simulink model "LAB_Triggred_SubSystem"  (R2024b)
settings: Solver=VariableStepAuto  StartTime=0.0  StopTime=10.0  RelTol=1e-3
settings Model: Creator=Ahmad  LastModifiedBy=Ahmad

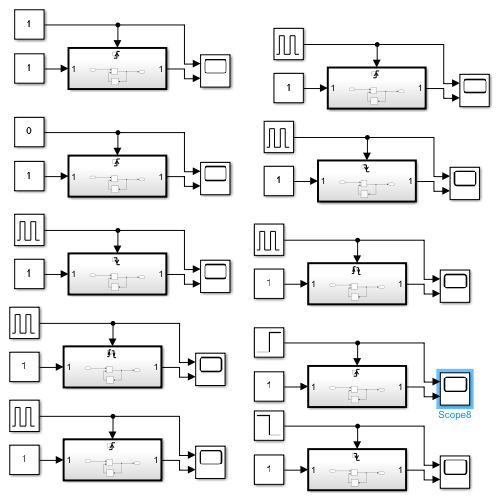
[thumbnail: Simulink's stored preview of the top-level diagram]
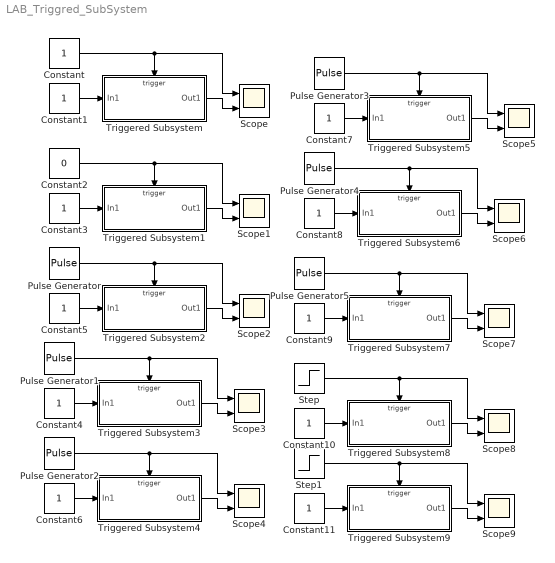
== system LAB_Triggred_SubSystem ==
  Constant{,1,3..11} (11 alike) : Constant
  Constant2 : Constant  Value=0
  Pulse Generator : DiscretePulseGenerator  PulseType=Time based  Period=10  PulseWidth=5
  Pulse Generator1 : DiscretePulseGenerator  PulseType=Time based  Amplitude=5  Period=10  PulseWidth=50
  Pulse Generator2 : DiscretePulseGenerator  PulseType=Time based  Amplitude=10  Period=10  PulseWidth=50  PhaseDelay=2
  Pulse Generator3 : DiscretePulseGenerator  PulseType=Time based  Amplitude=10  Period=1  PulseWidth=10
  Pulse Generator4 : DiscretePulseGenerator  PulseType=Time based  Amplitude=10  Period=1  PulseWidth=10
  Pulse Generator5 : DiscretePulseGenerator  PulseType=Time based  Amplitude=10  Period=1  PulseWidth=10
  Scope{,1..9} (10 alike) : Scope  NumInputPorts=2
  Step : Step  SampleTime=0
  Step1 : Step  Before=1  After=0  SampleTime=0
  Triggered Subsystem : Subsystem  TreatAsAtomicUnit=on
  Triggered Subsystem1 : Subsystem  TreatAsAtomicUnit=on
  Triggered Subsystem2 : Subsystem  TreatAsAtomicUnit=on
  Triggered Subsystem3 : Subsystem  TreatAsAtomicUnit=on
  Triggered Subsystem4 : Subsystem  TreatAsAtomicUnit=on
  Triggered Subsystem5 : Subsystem  TreatAsAtomicUnit=on
  Triggered Subsystem6 : Subsystem  TreatAsAtomicUnit=on
  Triggered Subsystem7 : Subsystem  TreatAsAtomicUnit=on
  Triggered Subsystem8 : Subsystem  TreatAsAtomicUnit=on
  Triggered Subsystem9 : Subsystem  TreatAsAtomicUnit=on
  wires:
  Constant/1 -> Scope/1, Triggered Subsystem/Trigger
  Constant1/1 -> Triggered Subsystem/1(In1)
  Triggered Subsystem/1(Out1) -> Scope/2
  Constant3/1 -> Triggered Subsystem1/1(In1)
  Constant2/1 -> Scope1/1, Triggered Subsystem1/Trigger
  Triggered Subsystem1/1(Out1) -> Scope1/2
  Pulse Generator/1 -> Scope2/1, Triggered Subsystem2/Trigger
  Triggered Subsystem2/1(Out1) -> Scope2/2
  Constant5/1 -> Triggered Subsystem2/1(In1)
  Pulse Generator1/1 -> Scope3/1, Triggered Subsystem3/Trigger
  Constant4/1 -> Triggered Subsystem3/1(In1)
  Triggered Subsystem3/1(Out1) -> Scope3/2
  Triggered Subsystem4/1(Out1) -> Scope4/2
  Constant6/1 -> Triggered Subsystem4/1(In1)
  Pulse Generator2/1 -> Scope4/1, Triggered Subsystem4/Trigger
  Triggered Subsystem5/1(Out1) -> Scope5/2
  Constant7/1 -> Triggered Subsystem5/1(In1)
  Pulse Generator3/1 -> Scope5/1, Triggered Subsystem5/Trigger
  Constant8/1 -> Triggered Subsystem6/1(In1)
  Pulse Generator4/1 -> Scope6/1, Triggered Subsystem6/Trigger
  Triggered Subsystem6/1(Out1) -> Scope6/2
  Constant9/1 -> Triggered Subsystem7/1(In1)
  Pulse Generator5/1 -> Scope7/1, Triggered Subsystem7/Trigger
  Triggered Subsystem7/1(Out1) -> Scope7/2
  Triggered Subsystem8/1(Out1) -> Scope8/2
  Step/1 -> Scope8/1, Triggered Subsystem8/Trigger
  Constant10/1 -> Triggered Subsystem8/1(In1)
  Constant11/1 -> Triggered Subsystem9/1(In1)
  Triggered Subsystem9/1(Out1) -> Scope9/2
  Step1/1 -> Scope9/1, Triggered Subsystem9/Trigger

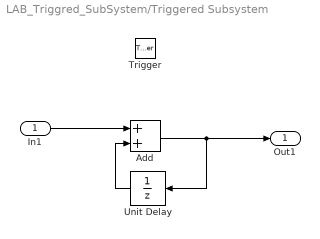
== system LAB_Triggred_SubSystem/Triggered Subsystem ==
  In1 : Inport
  Trigger : TriggerPort  VariantControl=(inherit)
  Add : Sum
  Unit Delay : UnitDelay  SampleTime=-1  HasFrameUpgradeWarning=on
  Out1 : Outport
  wires:
  In1/1 -> Add/1
  Add/1 -> Unit Delay/1, Out1/1
  Unit Delay/1 -> Add/2

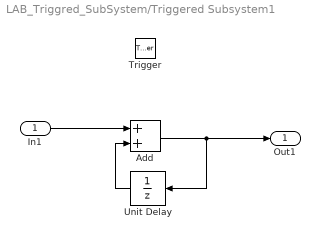
== system LAB_Triggred_SubSystem/Triggered Subsystem1 ==
  In1 : Inport
  Trigger : TriggerPort  VariantControl=(inherit)
  Add : Sum
  Unit Delay : UnitDelay  SampleTime=-1  HasFrameUpgradeWarning=on
  Out1 : Outport
  wires:
  In1/1 -> Add/1
  Add/1 -> Unit Delay/1, Out1/1
  Unit Delay/1 -> Add/2

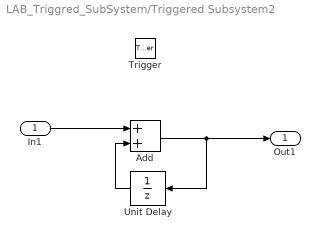
== system LAB_Triggred_SubSystem/Triggered Subsystem2 ==
  In1 : Inport
  Trigger : TriggerPort  TriggerType=falling  VariantControl=(inherit)
  Add : Sum
  Unit Delay : UnitDelay  SampleTime=-1  HasFrameUpgradeWarning=on
  Out1 : Outport
  wires:
  In1/1 -> Add/1
  Add/1 -> Unit Delay/1, Out1/1
  Unit Delay/1 -> Add/2

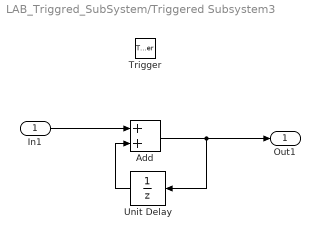
== system LAB_Triggred_SubSystem/Triggered Subsystem3 ==
  In1 : Inport
  Trigger : TriggerPort  TriggerType=either  VariantControl=(inherit)
  Add : Sum
  Unit Delay : UnitDelay  SampleTime=-1  HasFrameUpgradeWarning=on
  Out1 : Outport
  wires:
  In1/1 -> Add/1
  Add/1 -> Unit Delay/1, Out1/1
  Unit Delay/1 -> Add/2

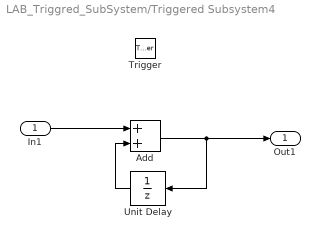
== system LAB_Triggred_SubSystem/Triggered Subsystem4 ==
  In1 : Inport
  Trigger : TriggerPort  VariantControl=(inherit)
  Add : Sum
  Unit Delay : UnitDelay  SampleTime=-1  HasFrameUpgradeWarning=on
  Out1 : Outport
  wires:
  In1/1 -> Add/1
  Add/1 -> Unit Delay/1, Out1/1
  Unit Delay/1 -> Add/2

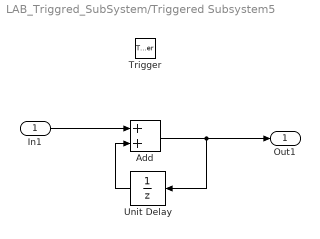
== system LAB_Triggred_SubSystem/Triggered Subsystem5 ==
  In1 : Inport
  Trigger : TriggerPort  VariantControl=(inherit)
  Add : Sum
  Unit Delay : UnitDelay  SampleTime=-1  HasFrameUpgradeWarning=on
  Out1 : Outport
  wires:
  In1/1 -> Add/1
  Add/1 -> Unit Delay/1, Out1/1
  Unit Delay/1 -> Add/2

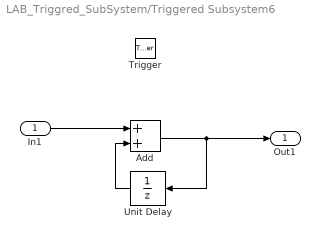
== system LAB_Triggred_SubSystem/Triggered Subsystem6 ==
  In1 : Inport
  Trigger : TriggerPort  TriggerType=falling  VariantControl=(inherit)
  Add : Sum
  Unit Delay : UnitDelay  SampleTime=-1  HasFrameUpgradeWarning=on
  Out1 : Outport
  wires:
  In1/1 -> Add/1
  Add/1 -> Unit Delay/1, Out1/1
  Unit Delay/1 -> Add/2

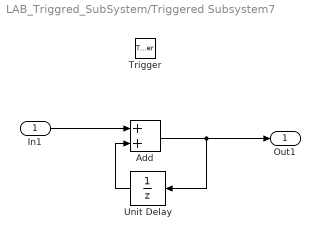
== system LAB_Triggred_SubSystem/Triggered Subsystem7 ==
  In1 : Inport
  Trigger : TriggerPort  TriggerType=either  VariantControl=(inherit)
  Add : Sum
  Unit Delay : UnitDelay  SampleTime=-1  HasFrameUpgradeWarning=on
  Out1 : Outport
  wires:
  In1/1 -> Add/1
  Add/1 -> Unit Delay/1, Out1/1
  Unit Delay/1 -> Add/2

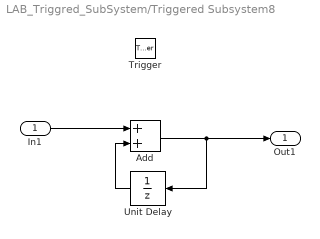
== system LAB_Triggred_SubSystem/Triggered Subsystem8 ==
  In1 : Inport
  Trigger : TriggerPort  VariantControl=(inherit)
  Add : Sum
  Unit Delay : UnitDelay  SampleTime=-1  HasFrameUpgradeWarning=on
  Out1 : Outport
  wires:
  In1/1 -> Add/1
  Add/1 -> Unit Delay/1, Out1/1
  Unit Delay/1 -> Add/2

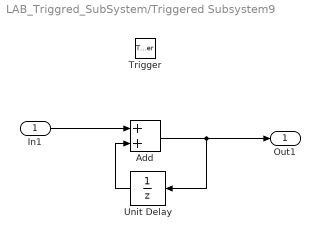
== system LAB_Triggred_SubSystem/Triggered Subsystem9 ==
  In1 : Inport
  Trigger : TriggerPort  TriggerType=falling  VariantControl=(inherit)
  Add : Sum
  Unit Delay : UnitDelay  SampleTime=-1  HasFrameUpgradeWarning=on
  Out1 : Outport
  wires:
  In1/1 -> Add/1
  Add/1 -> Unit Delay/1, Out1/1
  Unit Delay/1 -> Add/2
